simulink model "CAVE_MachE_driver_test"  (R2024a)
settings: configuration reference "ConfigSetDesktopFixedStep" (kept outside this file)
PreLoadFcn:
  | VSS_BICYCLE=Simulink.Variant('Dual=0');
  | VSS_DUAL=Simulink.Variant('Dual=1');
  | Dual=1;
  | load('DriveCycle2.mat')
PostLoadFcn:
  | if any(exist('dsrtsu_mdlpostloadfcn', 'file') ~= 0), dsrtsu_mdlpostloadfcn('Execute', bdroot); end
InitFcn:
  | , if any(exist('rtifpga_mdlclblib', 'file') ~= 0), rtifpga_mdlclblib('Init', bdroot); end,
  | , if any(exist('dsmpb_private', 'file') ~= 0), dsmpb_private('dsmpb_mdlclblib', 'Init', bdroot); end,
  | load('DriveCycle2.mat')
model workspace (MAT data in the model file):
  Gas = 0.383333333333
values from neighbouring files (symbols this model uses):
  CoastDown =     [Run_Simulink.mat]
  limitedMCT =     [Run_Simulink.mat]
  MCT =     [Run_Simulink.mat]
  optimized_speed = [6.8451519807e-19 6.71455685751e-19 6.61817305122e-19 6.79712455505e-19 6.66916107161e-19 6.93956205717e-19 6.71488581248e-19 6.61948887111e-19 6.81653289829e-19 6.68560882013e-19 6.9214695338e-19 6.73330729082e-19 ... (16417 elements, 16417x1)]    [OptimizedSpeed.mat]
  optimized_speed_time = [0 0.1 0.2 0.3 0.4 0.5 0.6 0.7 0.8 0.9 1 1.1 ... (16417 elements, 16417x1)]    [OptimizedSpeed.mat]
  pMCT =     [Run_Simulink.mat]
  RealSimPara =     [Run_Simulink.mat]
  Ref_speed = [13 13.007895099 13.015778396 13.023649891 13.031509584 13.039357475 13.047193564 13.055017851 13.062830336 13.070631019 13.0784199 13.086196979 ... (2669 elements, 2669x1)]    [Ref_speed_and_time.mat]
  Ref_time = [0 0.01 0.02 0.03 0.04 0.05 0.06 0.07 0.08 0.09 0.1 0.11 ... (2669 elements, 2669x1)]    [Ref_speed_and_time.mat]
  US06 =     [Run_Simulink.mat]
undefined symbols (not defined in the file or in its folder): AccelCmd, ActTqLF_Nm_, ActTqLR_Nm_, ActTqRF_Nm_, ActTqRR_Nm_, BattChargeLimitMaxPwr, BattChargeLimitSocBpts, BattChargeLimitTbl, BattChrgCapcty, BattDischargeLimitSocBpts, BattDischargeLimitTbl, BattDischargeMaxPwr, BattNumCellsParallel, BattNumCellsSeries, BattOpenVoltCapBpts, BattOpenVoltTbl, BattResistSocBpts, BattResistTbl, BattResistTempBpts, BrakeMaxPrs, BrakeMaxTrq, ChassisDistCg2FrontAxle, ChassisDistCg2RearAxle, ChassisVehMass, CltchCmd, DecelCmd, DiffRatio, DiscIntNeverNeededParam, EnvGravCnst, EnvPrs, EnvTemp, FuelSpecificGrav, GearCmd, h, InitStates, lgSw, MtrEffSpdBpts, MtrEffTbl, MtrEffTrqBpts, MtrPwrMax, MtrTrqMax, ResultsDrivingTests, SteeringCmd, SupvsryCtrlRegenBrkCutOffTbl, SupvsryCtrlRegenSpdBpts, TestScnrioCycleNum, VEH
libraries: simulink x122, VSIGenLib x122, etargetslib x75, dsmpblib x55, vehdynlibtire x24, autolibshared x22, CarMaker4SL x20, vehdynlibsuspension x14, vehdynlibtirecommon x14, autolibutils x10, VsrLibWheel x8, autolibpowerinfoutils x6
(part 16 of 32)

== system CAVE_MachE_driver_test/Vehicle Under Test3/Vehicle/Driver and Drive Cycle/Driver and PI with FF Control/Speed controller set/Predictive ==
  RefSpd [km/hr] : Inport
  In2 : Inport  Port=2
  Compare To Constant1 : simulink/Logic and Bit Operations/Compare To Constant  relop=<=  const=0.1  OutDataTypeStr=boolean  ZeroCross=off
  Constant : Constant  Value=0
  Constant1 : Constant  Value=0
  Gain : Gain  Gain=1/3.6
  Gain1 : Gain  Gain=1/3.6
  Gain4 : Gain  Gain=100
  Gain5 : Gain  Gain=100
  Longitudinal Driver : autolibshared/Longitudinal Driver  extAccelOvr=off  extDecelOvr=off  extAccelHld=off  extDecelHld=off  extAccelZero=off  extDecelZero=off  cntrlType=Predictive  shftType=None  velUnits=m/s  gearOut=off  Kp=10  Ki=5  Kff=.1  Kg=0  VehVelVec=[0 100]  KffVec=[.1 .1]  KpVec=[10 10]  KiVec=[5 5]  KgVec=[0 0]  m=2040  Kpt=6500  tau=0.1  L=3  aR=200/10  bR=2.5/100  cR=.3  g=9.807  vnom=5  Kaw=1  tauerr=.01  tauPt=2  GearInit=0  tShift=.1  pdlVec=[0.1 0.4 0.5 0.9]  upShftTbl=[-1 12.9375 26.4375 39.9375 51.18749999999999 62.4375 72.84375 83.25;-1 16.3125 29.8125 43.3125 54.5624 65.8125 76.78125 87.75;-1 19.6875 33.1875 46.68749999999999 57.9375 69.1875 80.71875 92.25;-1 33 52.5 77.25 100.5 138.75 161.875 185]  dwnShftTbl=[1 9.5625 23.0625 36.5625 47.8125 59.0625 68.90625 78.75;1 12.9375 26.4375 39.9375 51.18749999999999 62.4375 72.84375 83.25;1 16.3125 29.8125 43.3125 54.562499 65.8125 76.78125 87.75;1 19.6875 33.1875 46.68749999999999 57.9375 69.1875 80.71875 92.25]  tClutch=.5  tRev=.5  tPark=120  aMode=2  UpGearVec="[0  1  2  3  4  5  6  7]"  DownGearVec="[1  2  3  4  5  6  7  8]"
      settings: LibrarySourceBlock=vehdynlibdriver/Longitudinal Driver
  Lowpass Filter : TransferFcn  Denominator=[.02 1]
  Min threshold for Brake switch : Constant  Value=0
  Relational Operator : RelationalOperator  Operator=>  OutDataTypeStr=boolean  InputSameDT=off
  Switch3 : Switch  Criteria=u2 > Threshold  SaturateOnIntegerOverflow=off  InputSameDT=off
  Switch4 : Switch  Criteria=u2 > Threshold  SaturateOnIntegerOverflow=off  InputSameDT=off
  Terminator : Terminator
  standstill brake [0,1] : Constant  Value=0.5
  AccelPedalCmd : Outport
  BrakePedalCmd : Outport  Port=2
  Out3 : Outport  Port=3
  wires:
  Gain1/1 -> Longitudinal Driver/2
  Min threshold for Brake switch/1 -> Relational Operator/2
  Relational Operator/1 -> Out3/1  "BrakeSwitch"
  Constant1/1 -> Longitudinal Driver/3
  RefSpd [km/hr]/1 -> Gain/1
  In2/1 -> Lowpass Filter/1
  Longitudinal Driver/1 -> Terminator/1
  standstill brake [0,1]/1 -> Switch4/1
  Longitudinal Driver/3 -> Switch4/3, Relational Operator/1  "BrakePedalPosPre_pct"
  Switch4/1 -> Gain5/1  "BrakePedalPos_pct"
  Switch3/1 -> Gain4/1  "AcceleratorPedalPos_pct"
  Compare To Constant1/1 -> Switch4/2, Switch3/2
  Constant/1 -> Switch3/1
  Gain4/1 -> AccelPedalCmd/1  "AccelPedalCmd"
  Gain/1 -> Compare To Constant1/1, Longitudinal Driver/1
  Gain5/1 -> BrakePedalCmd/1  "BrakePedalCmd"
  Longitudinal Driver/2 -> Switch3/3  "AcceleratorPedalPosPre_pct"
  Lowpass Filter/1 -> Gain1/1  "VS_Flt"

== system CAVE_MachE_driver_test/Vehicle Under Test3/Vehicle/Driver and Drive Cycle/Driver and PI with FF Control/Speed controller set/Speed tracking controller ==
  RefSpd [km/hr] : Inport
  In2 : Inport  Port=2
  In-house CAVE : Subsystem  VariantControl=varaint1
  PIF : Subsystem  VariantControl=varaint2
  Predictive : Subsystem  VariantControl=varaint3
  AccelPedalCmd : Outport
  BrakePedalCmd : Outport  Port=2
  Out3 : Outport  Port=3

== system CAVE_MachE_driver_test/Vehicle Under Test3/Vehicle/Powertrain Supervisory Controller /Engine Torque Command/Accel Pedal to Traction Wheel Torque Request1/Max Motor Torque ==
  MtrSpd : Inport
  Constant : Constant  Value=MtrPwrMax
  Divide : Product  Inputs=*/
  Saturation : Saturate  UpperLimit=MtrTrqMax  LowerLimit=0
  Saturation1 : Saturate  UpperLimit=inf  LowerLimit=1
  MtrTrqMax : Outport
  wires:
  Saturation/1 -> MtrTrqMax/1
  Saturation1/1 -> Divide/2
  Divide/1 -> Saturation/1
  MtrSpd/1 -> Saturation1/1
  Constant/1 -> Divide/1

== system CAVE_MachE_driver_test/Vehicle Under Test3/Vehicle/Powertrain Supervisory Controller /Engine Torque Command/Motor Torque Arbitration and Power Management/Power Management ==
  note: Power Management algorithm:
      | - Estimate Elec power based on mech power using efficiency map
      | - Check if Elec power is within battery power limits
      | - If power within limit , use motor torque command
      | - If power limit exceeded, use limited motor torque
      | - For low Mot Spd, MotPwrReq will be a small number.  Pass through torque command until Mot Spd > 2.
  BattPwrDischrgLmt : Inport
  BattPwrChrgLmt : Inport  Port=2
  MotSpd : Inport  Port=3
  MotTrqCmd : Inport  Port=4
  Abs : Abs  SaturateOnIntegerOverflow=off
  Check Within Limits : Subsystem
  Compare To Constant : simulink/Logic and Bit Operations/Compare To Constant  relop=<  const=2  OutDataTypeStr=boolean
  ElecToMechPwr : Product  Inputs=*/
  Mech to Elec Power Estimate : Subsystem
  MechPwrToTrq : Product  Inputs=*/
  Switch : Switch  Criteria=u2 > Threshold  SaturateOnIntegerOverflow=off  InputSameDT=off
  Switch1 : Switch  Criteria=u2 > Threshold  SaturateOnIntegerOverflow=off  InputSameDT=off
  Torque Limit : Subsystem
  div0protect - poly : autolibutils/div0protect - poly  thresh=2  ZeroCross1=on  aMode=aMode
  MotTrqCmdFinal : Outport  VectorParamsAs1DForOutWhenUnconnected=off
  wires:
  Compare To Constant/1 -> Switch1/2
  Abs/1 -> Compare To Constant/1
  Switch1/1 -> Torque Limit/1(MotTrq)
  Check Within Limits/1(InLimit) -> Switch/2
  Switch/1 -> Switch1/3
  Check Within Limits/2(y) -> ElecToMechPwr/1
  BattPwrChrgLmt/1 -> Check Within Limits/3(lo)
  Mech to Elec Power Estimate/1(MotPwrElecReq) -> Check Within Limits/2(u)
  BattPwrDischrgLmt/1 -> Check Within Limits/1(up)
  Torque Limit/1(MotTrqCmd) -> MotTrqCmdFinal/1
  MechPwrToTrq/1 -> Switch/3
  ElecToMechPwr/1 -> MechPwrToTrq/1
  Mech to Elec Power Estimate/2(Eff2k) -> ElecToMechPwr/2
  div0protect - poly/1 -> MechPwrToTrq/2
  MotTrqCmd/1 -> Mech to Elec Power Estimate/1(MotTrqCmd), Switch1/1, Switch/1
  MotSpd/1 -> Abs/1, Mech to Elec Power Estimate/2(MotSpd), div0protect - poly/1, Torque Limit/2(MotSpd)

== system CAVE_MachE_driver_test/Vehicle Under Test3/Vehicle/Rototest and ORNL Interface/From Rototest/RotoTestEthRX/Depacker ==
  SysStsBits : Inport
  Extract Bits1 : simulink/Logic and Bit Operations/Extract Bits  bitsToExtract=Range of bits  numBits=8  bitIdxRange=[7]  outScalingMode=Preserve fixed-point scaling
  Extract Bits10 : simulink/Logic and Bit Operations/Extract Bits  bitsToExtract=Range of bits  numBits=8  bitIdxRange=[9]  outScalingMode=Preserve fixed-point scaling
  Extract Bits11 : simulink/Logic and Bit Operations/Extract Bits  bitsToExtract=Range of bits  numBits=8  bitIdxRange=[10]  outScalingMode=Preserve fixed-point scaling
  Extract Bits12 : simulink/Logic and Bit Operations/Extract Bits  bitsToExtract=Range of bits  numBits=8  bitIdxRange=[11]  outScalingMode=Preserve fixed-point scaling
  Extract Bits13 : simulink/Logic and Bit Operations/Extract Bits  bitsToExtract=Range of bits  numBits=8  bitIdxRange=[12]  outScalingMode=Preserve fixed-point scaling
  Extract Bits14 : simulink/Logic and Bit Operations/Extract Bits  bitsToExtract=Range of bits  numBits=8  bitIdxRange=[13]  outScalingMode=Preserve fixed-point scaling
  Extract Bits15 : simulink/Logic and Bit Operations/Extract Bits  bitsToExtract=Range of bits  numBits=8  bitIdxRange=[14]  outScalingMode=Preserve fixed-point scaling
  Extract Bits16 : simulink/Logic and Bit Operations/Extract Bits  bitsToExtract=Range of bits  numBits=8  bitIdxRange=[15]  outScalingMode=Preserve fixed-point scaling
  Extract Bits2 : simulink/Logic and Bit Operations/Extract Bits  bitsToExtract=Range of bits  numBits=8  bitIdxRange=[6]  outScalingMode=Preserve fixed-point scaling
  Extract Bits3 : simulink/Logic and Bit Operations/Extract Bits  bitsToExtract=Range of bits  numBits=8  bitIdxRange=[5]  outScalingMode=Preserve fixed-point scaling
  Extract Bits4 : simulink/Logic and Bit Operations/Extract Bits  bitsToExtract=Range of bits  numBits=8  bitIdxRange=[4]  outScalingMode=Preserve fixed-point scaling
  Extract Bits5 : simulink/Logic and Bit Operations/Extract Bits  bitsToExtract=Range of bits  numBits=8  bitIdxRange=[3]  outScalingMode=Preserve fixed-point scaling
  Extract Bits6 : simulink/Logic and Bit Operations/Extract Bits  bitsToExtract=Range of bits  numBits=8  bitIdxRange=[2]  outScalingMode=Preserve fixed-point scaling
  Extract Bits7 : simulink/Logic and Bit Operations/Extract Bits  bitsToExtract=Range of bits  numBits=8  bitIdxRange=[1]  outScalingMode=Preserve fixed-point scaling
  Extract Bits8 : simulink/Logic and Bit Operations/Extract Bits  bitsToExtract=Range of bits  numBits=8  bitIdxRange=[0]  outScalingMode=Preserve fixed-point scaling
  Extract Bits9 : simulink/Logic and Bit Operations/Extract Bits  bitsToExtract=Range of bits  numBits=8  bitIdxRange=[8]  outScalingMode=Preserve fixed-point scaling
  Gain : Gain  Gain=1/128
  Gain1 : Gain  Gain=1/64
  Gain10 : Gain  Gain=1/1024
  Gain11 : Gain  Gain=1/2048
  Gain12 : Gain  Gain=1/4096
  Gain13 : Gain  Gain=1/8192
  Gain14 : Gain  Gain=1/16384
  Gain15 : Gain  Gain=1/32768
  Gain2 : Gain  Gain=1/32
  Gain3 : Gain  Gain=1/16
  Gain4 : Gain  Gain=1/8
  Gain5 : Gain  Gain=1/4
  Gain6 : Gain  Gain=1/2
  Gain7 : Gain  Gain=1/1
  Gain8 : Gain  Gain=1/256
  Gain9 : Gain  Gain=1/512
  Header : VSIGenLib/Header  not=''
  Terminator{,1..8} (9 alike) : Terminator
  FaultActive : Outport
  WarningsActive : Outport  Port=2
  SpTqRR : Outport  Port=3
  SpTqLR : Outport  Port=4
  SpTqRF : Outport  Port=5
  SpTqLF : Outport  Port=6
  SystemActive : Outport  Port=7
  wires:
  Gain5/1 -> Terminator3/1  "Reserved"
  Gain6/1 -> Terminator4/1  "Reserved"
  Gain3/1 -> Terminator1/1  "Reserved"
  Gain4/1 -> Terminator2/1  "Reserved"
  Gain2/1 -> Terminator/1  "Reserved"
  Gain1/1 -> WarningsActive/1  "WarningsActive"
  Gain/1 -> FaultActive/1  "FaultActive"
  Gain7/1 -> Terminator5/1  "Reserved"
  Gain8/1 -> SystemActive/1  "SystemActive"
  Gain9/1 -> SpTqLF/1  "SpTqLF"
  Gain10/1 -> SpTqRF/1  "SpTqRF"
  Gain11/1 -> SpTqLR/1  "SpTqLR"
  Gain12/1 -> SpTqRR/1  "SpTqRR"
  Gain14/1 -> Terminator7/1  "Reserved"
  Gain13/1 -> Terminator8/1  "Reserved"
  Gain15/1 -> Terminator6/1  "Reserved"
  SysStsBits/1 -> Extract Bits9/1, Extract Bits10/1, Extract Bits16/1, Extract Bits15/1, Extract Bits14/1, Extract Bits13/1, Extract Bits12/1, Extract Bits11/1, Extract Bits8/1, Extract Bits7/1, Extract Bits6/1, Extract Bits5/1, Extract Bits4/1, Extract Bits3/1, Extract Bits2/1, Extract Bits1/1
  Extract Bits16/1 -> Gain15/1
  Extract Bits14/1 -> Gain13/1
  Extract Bits15/1 -> Gain14/1
  Extract Bits13/1 -> Gain12/1
  Extract Bits12/1 -> Gain11/1
  Extract Bits11/1 -> Gain10/1
  Extract Bits9/1 -> Gain8/1
  Extract Bits10/1 -> Gain9/1
  Extract Bits2/1 -> Gain1/1
  Extract Bits5/1 -> Gain4/1
  Extract Bits1/1 -> Gain/1
  Extract Bits3/1 -> Gain2/1
  Extract Bits7/1 -> Gain6/1
  Extract Bits8/1 -> Gain7/1
  Extract Bits4/1 -> Gain3/1
  Extract Bits6/1 -> Gain5/1

== system CAVE_MachE_driver_test/Vehicle Under Test3/Vehicle/Rototest and ORNL Interface/Get Wheel Spd Cmd Based on Wheel Dynamics/Whl Dynamics & Format CM Powertrain Signal/Diff Trq ==
  In1 : Inport
  Constant : Constant  Value=4.1
  Gain10 : Gain  Gain=0.5
  Product : Product  RndMeth=Zero
  Out1 : Outport
  wires:
  Gain10/1 -> Out1/1
  Constant/1 -> Product/1
  In1/1 -> Product/2
  Product/1 -> Gain10/1  "DiffTrq"

== system CAVE_MachE_driver_test/Vehicle Under Test3/Vehicle/Rototest and ORNL Interface/Get Wheel Spd Cmd Based on Wheel Dynamics/Whl Dynamics & Format CM Powertrain Signal/Subsystem ==
  BrakeTorq : Inport
  <Car Trq_T2WFL> : Inport  Port=2
  AxlTorq : Inport  Port=3
  Fx : Inport  Port=4
  Add1 : Sum  Inputs=--+
  Add2 : Sum  Inputs=-+
  Constant : Constant  Value=0
  Constant9 : Constant  Value=0.3135
  MATLAB Function : MATLAB Function  TreatAsAtomicUnit=on
  Memory : Memory
  Output Damping : Gain  Gain=0  SaturateOnIntegerOverflow=on  OutDataTypeStr=Inherit: Same as input  ParamDataTypeStr=Inherit: Same as input
  Product3 : Product  Inputs=**
  Saturation : Saturate  UpperLimit=inf  LowerLimit=0  ZeroCross=off
  Sum : Sum  Inputs=--
  Sum3 : Sum  Inputs=-++
  Switch : Switch  Criteria=u2 > Threshold  SaturateOnIntegerOverflow=off  InputSameDT=off
  WheelInertia : Subsystem
  WheelInertia1 : Subsystem
  omega wheel : Integrator  ContinuousStateAttributes='omegaWheel'
  rotv FL : Outport
  wires:
  Sum3/1 -> WheelInertia/1(In1)
  BrakeTorq/1 -> Sum3/1
  MATLAB Function/1(switchFlag) -> Switch/2  "Flag1"
  Constant/1 -> Switch/1
  Memory/1 -> MATLAB Function/2(wheelSpd)
  Add2/1 -> Saturation/1
  [RhoZ1] -> Add2/1
  Constant9/1 -> Add2/2
  AxlTorq/1 -> Add1/1, MATLAB Function/1(axleTorq), Sum3/3
  <Car Trq_T2WFL>/1 -> Add1/2, Sum3/2
  Product3/1 -> Add1/3
  Saturation/1 -> Product3/2
  Add1/1 -> WheelInertia1/1(In1)
  Switch/1 -> omega wheel/1
  omega wheel/1 -> Memory/1, Output Damping/1, rotv FL/1
  Output Damping/1 -> Sum/2
  WheelInertia1/1(axleTorq) -> Sum/1  "rota"
  Sum/1 -> Switch/3
  [Fx1] -> Product3/1

== system CAVE_MachE_driver_test/Vehicle Under Test3/Vehicle/Rototest and ORNL Interface/Get Wheel Spd Cmd Based on Wheel Dynamics/Whl Dynamics & Format CM Powertrain Signal/Subsystem1 ==
  BrakeTorq : Inport
  <Car Trq_T2WFL> : Inport  Port=2
  AxlTorq : Inport  Port=3
  Discrete-Time Integrator : DiscreteIntegrator  IntegratorMethod=Integration: Backward Euler  InitialCondition=0/3.6/0.3235  SampleTime=0.001  ICPrevOutput=DiscIntNeverNeededParam  ICPrevScaledInput=DiscIntNeverNeededParam
  Sum3 : Sum  Inputs=-++
  WheelInertia : Subsystem
  rotv FL : Outport
  wires:
  Sum3/1 -> WheelInertia/1(In1)
  AxlTorq/1 -> Sum3/3
  <Car Trq_T2WFL>/1 -> Sum3/2
  BrakeTorq/1 -> Sum3/1
  Discrete-Time Integrator/1 -> rotv FL/1  "rotv FL"
  WheelInertia/1(Out1) -> Discrete-Time Integrator/1

== system CAVE_MachE_driver_test/Vehicle Under Test3/Vehicle/Rototest and ORNL Interface/Get Wheel Spd Cmd Based on Wheel Dynamics/Whl Dynamics & Format CM Powertrain Signal/Subsystem2 ==
  BrakeTorq : Inport
  <Car Trq_T2WFR> : Inport  Port=2
  AxlTorq : Inport  Port=3
  Fx : Inport  Port=4
  Add1 : Sum  Inputs=--+
  Add2 : Sum  Inputs=-+
  Constant : Constant  Value=0
  Constant9 : Constant  Value=0.3135
  MATLAB Function : MATLAB Function  TreatAsAtomicUnit=on
  Memory : Memory
  Output Damping : Gain  Gain=-1  SaturateOnIntegerOverflow=on  OutDataTypeStr=Inherit: Same as input  ParamDataTypeStr=Inherit: Same as input
  Product3 : Product  Inputs=**
  Saturation : Saturate  UpperLimit=inf  LowerLimit=0  ZeroCross=off
  Sum3 : Sum  Inputs=-++
  Switch : Switch  Criteria=u2 > Threshold  SaturateOnIntegerOverflow=off  InputSameDT=off
  WheelInertia : Subsystem
  WheelInertia1 : Subsystem
  omega wheel : Integrator  ContinuousStateAttributes='omegaWheel'
  rotv FR : Outport
  wires:
  MATLAB Function/1(switchFlag) -> Switch/2
  Constant/1 -> Switch/1
  BrakeTorq/1 -> Sum3/1
  Sum3/1 -> WheelInertia/1(In1)
  Memory/1 -> MATLAB Function/2(wheelSpd)
  WheelInertia1/1(Out1) -> Output Damping/1  "rota"
  Product3/1 -> Add1/3
  <Car Trq_T2WFR>/1 -> Add1/2, Sum3/2
  Constant9/1 -> Add2/2
  Add1/1 -> WheelInertia1/1(In1)
  [RhoZ2] -> Add2/1
  Saturation/1 -> Product3/2
  Add2/1 -> Saturation/1
  AxlTorq/1 -> Add1/1, MATLAB Function/1(axleTorq), Sum3/3
  omega wheel/1 -> Memory/1, rotv FR/1
  Switch/1 -> omega wheel/1
  Output Damping/1 -> Switch/3
  [Fx2] -> Product3/1

== system CAVE_MachE_driver_test/Vehicle Under Test3/Vehicle/Rototest and ORNL Interface/Get Wheel Spd Cmd Based on Wheel Dynamics/Whl Dynamics & Format CM Powertrain Signal/Subsystem3 ==
  BrakeTorq : Inport
  <Car Trq_T2WRL> : Inport  Port=2
  AxlTorq : Inport  Port=3
  Fx : Inport  Port=4
  FWSpd : Inport  Port=5
  Add1 : Sum  Inputs=--+
  Add2 : Sum  Inputs=-+
  Constant : Constant  Value=0
  Constant9 : Constant  Value=0.3135
  MATLAB Function : MATLAB Function  TreatAsAtomicUnit=on
  Memory : Memory
  Output Damping : Gain  Gain=0  SaturateOnIntegerOverflow=on  OutDataTypeStr=Inherit: Same as input  ParamDataTypeStr=Inherit: Same as input
  Product3 : Product  Inputs=**
  Saturation : Saturate  UpperLimit=inf  LowerLimit=0  ZeroCross=off
  Sum : Sum  Inputs=--
  Sum3 : Sum  Inputs=-++
  Switch : Switch  Criteria=u2 > Threshold  SaturateOnIntegerOverflow=off  InputSameDT=off
  WheelInertia : Subsystem
  WheelInertia1 : Subsystem
  omega wheel : Integrator  ContinuousStateAttributes='omegaWheel'
  rotv RL : Outport
  wires:
  MATLAB Function/1(switchFlag) -> Switch/2
  Constant/1 -> Switch/1
  BrakeTorq/1 -> Sum3/1
  Sum3/1 -> WheelInertia/1(In1)
  Product3/1 -> Add1/3
  <Car Trq_T2WRL>/1 -> Sum3/2, Add1/2
  Constant9/1 -> Add2/2
  Add1/1 -> WheelInertia1/1(In1)
  [RhoZ3] -> Add2/1
  Saturation/1 -> Product3/2
  Add2/1 -> Saturation/1
  AxlTorq/1 -> Add1/1, MATLAB Function/1(axleTorq), Sum3/3
  FWSpd/1 -> MATLAB Function/2(wheelSpd)
  Sum/1 -> Switch/3
  Switch/1 -> omega wheel/1
  [Fx3] -> Product3/1
  Output Damping/1 -> Sum/2
  omega wheel/1 -> Output Damping/1, rotv RL/1
  WheelInertia1/1(axleTorq) -> Sum/1  "rota"

== system CAVE_MachE_driver_test/Vehicle Under Test3/Vehicle/Rototest and ORNL Interface/Get Wheel Spd Cmd Based on Wheel Dynamics/Whl Dynamics & Format CM Powertrain Signal/Subsystem4 ==
  BrakeTorq : Inport
  <Car Trq_T2WRR> : Inport  Port=2
  AxlTorq : Inport  Port=3
  Fx : Inport  Port=4
  FWSpd : Inport  Port=5
  Add1 : Sum  Inputs=--+
  Add2 : Sum  Inputs=-+
  Constant : Constant  Value=0
  Constant9 : Constant  Value=0.3135
  Gain : Gain  Gain=-1
  MATLAB Function : MATLAB Function  TreatAsAtomicUnit=on
  Memory : Memory
  Product3 : Product  Inputs=**
  Saturation : Saturate  UpperLimit=inf  LowerLimit=0  ZeroCross=off
  Sum3 : Sum  Inputs=-++
  Switch : Switch  Criteria=u2 > Threshold  SaturateOnIntegerOverflow=off  InputSameDT=off
  WheelInertia : Subsystem
  WheelInertia1 : Subsystem
  omega wheel : Integrator  ContinuousStateAttributes='omegaWheel'
  rotv RR : Outport
  wires:
  MATLAB Function/1(switchFlag) -> Switch/2
  Constant/1 -> Switch/1
  BrakeTorq/1 -> Sum3/1
  Sum3/1 -> WheelInertia/1(In1)
  Product3/1 -> Add1/3
  <Car Trq_T2WRR>/1 -> Add1/2, Sum3/2
  Constant9/1 -> Add2/2
  Add1/1 -> WheelInertia1/1(In1)
  [RhoZ4] -> Add2/1
  Saturation/1 -> Product3/2
  Add2/1 -> Saturation/1
  AxlTorq/1 -> Add1/1, MATLAB Function/1(axleTorq), Sum3/3
  FWSpd/1 -> MATLAB Function/2(wheelSpd)
  Gain/1 -> Switch/3
  Switch/1 -> omega wheel/1
  omega wheel/1 -> rotv RR/1
  [Fx4] -> Product3/1
  WheelInertia1/1(axleTorq) -> Gain/1  "rota"

== system CAVE_MachE_driver_test/Vehicle Under Test3/Vehicle/Rototest and ORNL Interface/Get Wheel Spd Cmd Based on Wheel Dynamics/Whl Dynamics & Format CM Powertrain Signal/Subsystem5 ==
  In1 : Inport
  <Car Trq_T2WFR> : Inport  Port=2
  In3 : Inport  Port=3
  Discrete-Time Integrator1 : DiscreteIntegrator  IntegratorMethod=Integration: Backward Euler  InitialCondition=0/3.6/0.3235  SampleTime=0.001  ICPrevOutput=DiscIntNeverNeededParam  ICPrevScaledInput=DiscIntNeverNeededParam
  Sum2 : Sum  Inputs=-++
  WheelInertia1 : Subsystem
  rotv FR : Outport
  wires:
  <Car Trq_T2WFR>/1 -> Sum2/2
  Sum2/1 -> WheelInertia1/1(In1)
  In3/1 -> Sum2/3
  WheelInertia1/1(Out1) -> Discrete-Time Integrator1/1  "rota"
  In1/1 -> Sum2/1
  Discrete-Time Integrator1/1 -> rotv FR/1  "rotv FR"

== system CAVE_MachE_driver_test/Vehicle Under Test3/Vehicle/Rototest and ORNL Interface/Get Wheel Spd Cmd Based on Wheel Dynamics/Whl Dynamics & Format CM Powertrain Signal/Subsystem6 ==
  In1 : Inport
  <Car Trq_T2WRL> : Inport  Port=2
  In3 : Inport  Port=3
  Discrete-Time Integrator2 : DiscreteIntegrator  IntegratorMethod=Integration: Backward Euler  InitialCondition=0/3.6/0.3235  SampleTime=0.001  ICPrevOutput=DiscIntNeverNeededParam  ICPrevScaledInput=DiscIntNeverNeededParam
  Sum : Sum  Inputs=-++
  WheelInertia2 : Subsystem
  rotv RL : Outport
  wires:
  In3/1 -> Sum/3
  WheelInertia2/1(Out1) -> Discrete-Time Integrator2/1  "rota"
  <Car Trq_T2WRL>/1 -> Sum/2
  Sum/1 -> WheelInertia2/1(In1)
  Discrete-Time Integrator2/1 -> rotv RL/1  "rotv RL"
  In1/1 -> Sum/1

== system CAVE_MachE_driver_test/Vehicle Under Test3/Vehicle/Rototest and ORNL Interface/Get Wheel Spd Cmd Based on Wheel Dynamics/Whl Dynamics & Format CM Powertrain Signal/Subsystem7 ==
  In1 : Inport
  <Car Trq_T2WRR> : Inport  Port=2
  In3 : Inport  Port=3
  Discrete-Time Integrator3 : DiscreteIntegrator  IntegratorMethod=Integration: Backward Euler  InitialCondition=0/3.6/0.3235  SampleTime=0.001  ICPrevOutput=DiscIntNeverNeededParam  ICPrevScaledInput=DiscIntNeverNeededParam
  Sum1 : Sum  Inputs=-++
  WheelInertia3 : Subsystem
  rotv RR : Outport
  wires:
  Sum1/1 -> WheelInertia3/1(In1)
  WheelInertia3/1(Out1) -> Discrete-Time Integrator3/1  "rota"
  In3/1 -> Sum1/3
  <Car Trq_T2WRR>/1 -> Sum1/2
  In1/1 -> Sum1/1
  Discrete-Time Integrator3/1 -> rotv RR/1  "rotv RR"

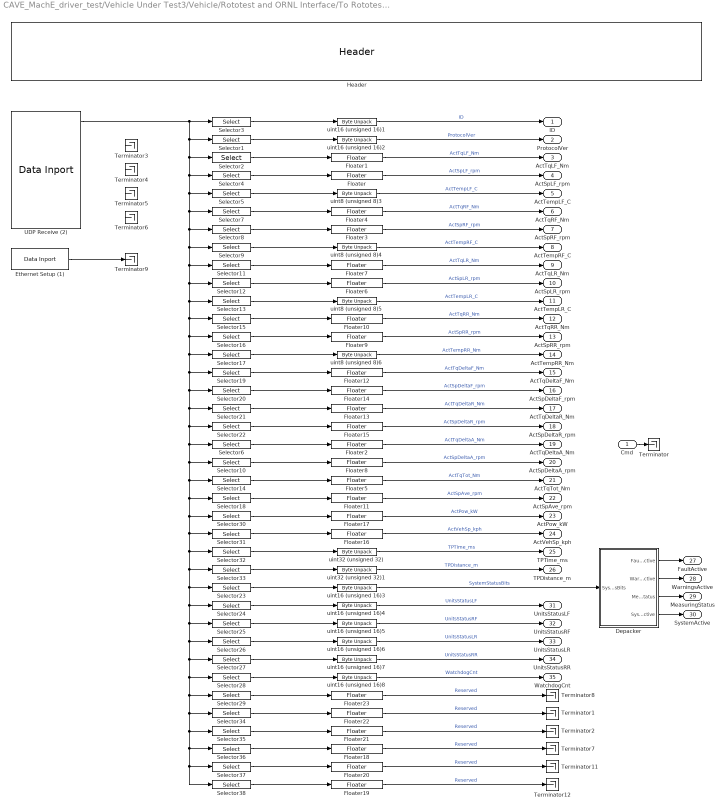
== system CAVE_MachE_driver_test/Vehicle Under Test3/Vehicle/Rototest and ORNL Interface/To Rototest with Band-Aid/Logging/RotoTestEthRXLogging ==
  Cmd : Inport
  Depacker : Subsystem
  Ethernet Setup (1) : dsmpblib/Data Inport  Priority=10000
      settings: SourceProductName=dSPACE Model Interface Package for Simulink (MIPS)
  Floater{,1..23} (24 alike) : VSIGenLib/Floater  SystemSampleTime=-1  VariantActivationTime=update diagram  AllowFlexibleInterface=on  Latency=0  AutoFrameSizeCalculation=off
  Header : VSIGenLib/Header  not=''
  Selector1 : Selector  IndexMode=Zero-based  InputPortWidth=124  IndexOptions=Index vector (dialog)  Indices=[3 2]  OutputSizes=1
  Selector10 : Selector  IndexMode=Zero-based  InputPortWidth=124  IndexOptions=Index vector (dialog)  Indices=[63 62 61 60]  OutputSizes=1
  Selector11 : Selector  IndexMode=Zero-based  InputPortWidth=124  IndexOptions=Index vector (dialog)  Indices=[25 24 23 22]  OutputSizes=1
  Selector12 : Selector  IndexMode=Zero-based  InputPortWidth=124  IndexOptions=Index vector (dialog)  Indices=[29 28 27 26]  OutputSizes=1
  Selector13 : Selector  IndexMode=Zero-based  InputPortWidth=124  IndexOptions=Index vector (dialog)  Indices=[30]  OutputSizes=1
  Selector14 : Selector  IndexMode=Zero-based  InputPortWidth=124  IndexOptions=Index vector (dialog)  Indices=[67 66 65 64]  OutputSizes=1
  Selector15 : Selector  IndexMode=Zero-based  InputPortWidth=124  IndexOptions=Index vector (dialog)  Indices=[34 33 32 31]  OutputSizes=1
  Selector16 : Selector  IndexMode=Zero-based  InputPortWidth=124  IndexOptions=Index vector (dialog)  Indices=[38 37 36 35]  OutputSizes=1
  Selector17 : Selector  IndexMode=Zero-based  InputPortWidth=124  IndexOptions=Index vector (dialog)  Indices=[39]  OutputSizes=1
  Selector18 : Selector  IndexMode=Zero-based  InputPortWidth=124  IndexOptions=Index vector (dialog)  Indices=[71 70 69 68]  OutputSizes=1
  Selector19 : Selector  IndexMode=Zero-based  InputPortWidth=124  IndexOptions=Index vector (dialog)  Indices=[43 42 41 40]  OutputSizes=1
  Selector2 : Selector  IndexMode=Zero-based  InputPortWidth=124  IndexOptions=Index vector (dialog)  Indices=[7 6 5 4]  OutputSizes=1
  Selector20 : Selector  IndexMode=Zero-based  InputPortWidth=124  IndexOptions=Index vector (dialog)  Indices=[47 46 45 44]  OutputSizes=1
  Selector21 : Selector  IndexMode=Zero-based  InputPortWidth=124  IndexOptions=Index vector (dialog)  Indices=[51 50 49 48]  OutputSizes=1
  Selector22 : Selector  IndexMode=Zero-based  InputPortWidth=124  IndexOptions=Index vector (dialog)  Indices=[55 54 53 52]  OutputSizes=1
  Selector23 : Selector  IndexMode=Zero-based  InputPortWidth=124  IndexOptions=Index vector (dialog)  Indices=[89 88]  OutputSizes=1
  Selector24 : Selector  IndexMode=Zero-based  InputPortWidth=124  IndexOptions=Index vector (dialog)  Indices=[91 90]  OutputSizes=1
  Selector25 : Selector  IndexMode=Zero-based  InputPortWidth=124  IndexOptions=Index vector (dialog)  Indices=[93 92]  OutputSizes=1
  Selector26 : Selector  IndexMode=Zero-based  InputPortWidth=124  IndexOptions=Index vector (dialog)  Indices=[95 94]  OutputSizes=1
  Selector27 : Selector  IndexMode=Zero-based  InputPortWidth=124  IndexOptions=Index vector (dialog)  Indices=[97 96]  OutputSizes=1
  Selector28 : Selector  IndexMode=Zero-based  InputPortWidth=124  IndexOptions=Index vector (dialog)  Indices=[99 98]  OutputSizes=1
  Selector29 : Selector  IndexMode=Zero-based  InputPortWidth=124  IndexOptions=Index vector (dialog)  Indices=[103 102 101 100]  OutputSizes=1
  Selector3 : Selector  IndexMode=Zero-based  InputPortWidth=124  IndexOptions=Index vector (dialog)  Indices=[1 0]  OutputSizes=1
  Selector30 : Selector  IndexMode=Zero-based  InputPortWidth=124  IndexOptions=Index vector (dialog)  Indices=[67 66 65 64]  OutputSizes=1
  Selector31 : Selector  IndexMode=Zero-based  InputPortWidth=124  IndexOptions=Index vector (dialog)  Indices=[71 70 69 68]  OutputSizes=1
  Selector32 : Selector  IndexMode=Zero-based  InputPortWidth=124  IndexOptions=Index vector (dialog)  Indices=[83 82 81 80]  OutputSizes=1
  Selector33 : Selector  IndexMode=Zero-based  InputPortWidth=124  IndexOptions=Index vector (dialog)  Indices=[87 86 85 84]  OutputSizes=1
  Selector34 : Selector  IndexMode=Zero-based  InputPortWidth=124  IndexOptions=Index vector (dialog)  Indices=[107 106 105 104]  OutputSizes=1
  Selector35 : Selector  IndexMode=Zero-based  InputPortWidth=124  IndexOptions=Index vector (dialog)  Indices=[111 110 109 108]  OutputSizes=1
  Selector36 : Selector  IndexMode=Zero-based  InputPortWidth=124  IndexOptions=Index vector (dialog)  Indices=[115 114 113 112]  OutputSizes=1
  Selector37 : Selector  IndexMode=Zero-based  InputPortWidth=124  IndexOptions=Index vector (dialog)  Indices=[119 118 117 116]  OutputSizes=1
  Selector38 : Selector  IndexMode=Zero-based  InputPortWidth=124  IndexOptions=Index vector (dialog)  Indices=[123 122 121 120]  OutputSizes=1
  Selector4 : Selector  IndexMode=Zero-based  InputPortWidth=124  IndexOptions=Index vector (dialog)  Indices=[11 10 9 8]  OutputSizes=1
  Selector5 : Selector  IndexMode=Zero-based  InputPortWidth=124  IndexOptions=Index vector (dialog)  Indices=[12]  OutputSizes=1
  Selector6 : Selector  IndexMode=Zero-based  InputPortWidth=124  IndexOptions=Index vector (dialog)  Indices=[59 58 57 56]  OutputSizes=1
  Selector7 : Selector  IndexMode=Zero-based  InputPortWidth=124  IndexOptions=Index vector (dialog)  Indices=[16 15 14 13]  OutputSizes=1
  Selector8 : Selector  IndexMode=Zero-based  InputPortWidth=124  IndexOptions=Index vector (dialog)  Indices=[20 19 18 17]  OutputSizes=1
  Selector9 : Selector  IndexMode=Zero-based  InputPortWidth=124  IndexOptions=Index vector (dialog)  Indices=[21]  OutputSizes=1
  Terminator{,1..9,11..12} (12 alike) : Terminator
  UDP Receive (2) : dsmpblib/Data Inport  Priority=10000
      settings: SourceProductName=dSPACE Model Interface Package for Simulink (MIPS)
  uint16 (unsigned 16){1..8} (8 alike) : etargetslib/Byte Unpack  dimensions={[1]}  datatypes={'uint16'}  byteAlign=1
  uint32 (unsigned 32) : etargetslib/Byte Unpack  dimensions={[1]}  datatypes={'uint32'}  byteAlign=1
  uint32 (unsigned 32)1 : etargetslib/Byte Unpack  dimensions={[1]}  datatypes={'uint32'}  byteAlign=1
  uint8 (unsigned 8){3..6} (4 alike) : etargetslib/Byte Unpack  dimensions={[1]}  datatypes={'uint8'}  byteAlign=1
  ID : Outport
  ProtocolVer : Outport  Port=2
  ActTqLF_Nm : Outport  Port=3
  ActSpLF_rpm : Outport  Port=4
  ActTempLF_C : Outport  Port=5
  ActTqRF_Nm : Outport  Port=6
  ActSpRF_rpm : Outport  Port=7
  ActTempRF_C : Outport  Port=8
  ActTqLR_Nm : Outport  Port=9
  ActSpLR_rpm : Outport  Port=10
  ActTempLR_C : Outport  Port=11
  ActTqRR_Nm : Outport  Port=12
  ActSpRR_rpm : Outport  Port=13
  ActTempRR_Nm : Outport  Port=14
  ActTqDeltaF_Nm : Outport  Port=15
  ActSpDeltaF_rpm : Outport  Port=16
  ActTqDeltaR_Nm : Outport  Port=17
  ActSpDeltaR_rpm : Outport  Port=18
  ActTqDeltaA_Nm : Outport  Port=19
  ActSpDeltaA_rpm : Outport  Port=20
  ActTqTot_Nm : Outport  Port=21
  ActSpAve_rpm : Outport  Port=22
  ActPow_kW : Outport  Port=23
  ActVehSp_kph : Outport  Port=24
  TPTime_ms : Outport  Port=25
  TPDistance_m : Outport  Port=26
  FaultActive : Outport  Port=27
  WarningsActive : Outport  Port=28
  MeasuringStatus : Outport  Port=29
  SystemActive : Outport  Port=30
  UnitsStatusLF : Outport  Port=31
  UnitsStatusRF : Outport  Port=32
  UnitsStatusLR : Outport  Port=33
  UnitsStatusRR : Outport  Port=34
  WatchdogCnt : Outport  Port=35
  wires:
  Selector11/1 -> Floater7/1
  Floater10/1 -> ActTqRR_Nm/1  "ActTqRR_Nm"
  Selector4/1 -> Floater/1
  ? -> Terminator6/1
  Selector1/1 -> uint16 (unsigned 16)2/1
  Selector19/1 -> Floater12/1
  Selector21/1 -> Floater13/1
  Selector28/1 -> uint16 (unsigned 16)8/1
  ? -> Terminator5/1
  Selector3/1 -> uint16 (unsigned 16)1/1
  uint8 (unsigned 8)5/1 -> ActTempLR_C/1  "ActTempLR_C"
  Selector16/1 -> Floater9/1
  Selector15/1 -> Floater10/1
  Selector5/1 -> uint8 (unsigned 8)3/1
  Selector9/1 -> uint8 (unsigned 8)4/1
  Selector20/1 -> Floater14/1
  Floater6/1 -> ActSpLR_rpm/1  "ActSpLR_rpm"
  uint8 (unsigned 8)6/1 -> ActTempRR_Nm/1  "ActTempRR_Nm"
  Selector29/1 -> Floater23/1
  Floater4/1 -> ActTqRF_Nm/1  "ActTqRF_Nm"
  Selector25/1 -> uint16 (unsigned 16)5/1
  ? -> Terminator3/1
  Floater3/1 -> ActSpRF_rpm/1  "ActSpRF_rpm"
  uint16 (unsigned 16)3/1 -> Depacker/1(SysStsBits)  "SystemStatusBits"
  Selector26/1 -> uint16 (unsigned 16)6/1
  Selector13/1 -> uint8 (unsigned 8)5/1
  Selector2/1 -> Floater1/1
  Floater13/1 -> ActTqDeltaR_Nm/1  "ActTqDeltaR_Nm"
  Selector27/1 -> uint16 (unsigned 16)7/1
  uint16 (unsigned 16)4/1 -> UnitsStatusLF/1  "UnitsStatusLF"
  ? -> Terminator4/1
  Selector17/1 -> uint8 (unsigned 8)6/1
  uint16 (unsigned 16)6/1 -> UnitsStatusLR/1  "UnitsStatusLR"
  Selector23/1 -> uint16 (unsigned 16)3/1
  Selector12/1 -> Floater6/1
  Selector22/1 -> Floater15/1
  uint16 (unsigned 16)7/1 -> UnitsStatusRR/1  "UnitsStatusRR"
  Selector8/1 -> Floater3/1
  Selector7/1 -> Floater4/1
  Selector24/1 -> uint16 (unsigned 16)4/1
  uint16 (unsigned 16)2/1 -> ProtocolVer/1  "ProtocolVer"
  Floater7/1 -> ActTqLR_Nm/1  "ActTqLR_Nm"
  Floater12/1 -> ActTqDeltaF_Nm/1  "ActTqDeltaF_Nm"
  uint8 (unsigned 8)3/1 -> ActTempLF_C/1  "ActTempLF_C"
  Floater1/1 -> ActTqLF_Nm/1  "ActTqLF_Nm"
  Floater9/1 -> ActSpRR_rpm/1  "ActSpRR_rpm"
  uint16 (unsigned 16)5/1 -> UnitsStatusRF/1  "UnitsStatusRF"
  Floater14/1 -> ActSpDeltaF_rpm/1  "ActSpDeltaF_rpm"
  uint16 (unsigned 16)8/1 -> WatchdogCnt/1  "WatchdogCnt"
  Floater15/1 -> ActSpDeltaR_rpm/1  "ActSpDeltaR_rpm"
  uint16 (unsigned 16)1/1 -> ID/1  "ID"
  Floater/1 -> ActSpLF_rpm/1  "ActSpLF_rpm"
  uint8 (unsigned 8)4/1 -> ActTempRF_C/1  "ActTempRF_C"
  Depacker/3(MeasuringStatus) -> MeasuringStatus/1
  Depacker/2(WarningsActive) -> WarningsActive/1
  Depacker/1(FaultActive) -> FaultActive/1
  Depacker/4(SystemActive) -> SystemActive/1
  Ethernet Setup (1)/1 -> Terminator9/1
  Floater11/1 -> ActSpAve_rpm/1  "ActSpAve_rpm"
  Floater8/1 -> ActSpDeltaA_rpm/1  "ActSpDeltaA_rpm"
  Floater2/1 -> ActTqDeltaA_Nm/1  "ActTqDeltaA_Nm"
  Selector18/1 -> Floater11/1
  Floater5/1 -> ActTqTot_Nm/1  "ActTqTot_Nm"
  Selector10/1 -> Floater8/1
  Selector14/1 -> Floater5/1
  Selector6/1 -> Floater2/1
  Selector30/1 -> Floater17/1
  Floater17/1 -> ActPow_kW/1  "ActPow_kW"
  Selector31/1 -> Floater16/1
  Floater16/1 -> ActVehSp_kph/1  "ActVehSp_kph"
  uint32 (unsigned 32)/1 -> TPTime_ms/1  "TPTime_ms"
  uint32 (unsigned 32)1/1 -> TPDistance_m/1  "TPDistance_m"
  Selector33/1 -> uint32 (unsigned 32)1/1
  Selector32/1 -> uint32 (unsigned 32)/1
  Selector34/1 -> Floater22/1
  Selector35/1 -> Floater21/1
  Selector36/1 -> Floater18/1
  Selector37/1 -> Floater20/1
  UDP Receive (2)/1 -> Selector3/1, Selector1/1, Selector2/1, Selector4/1, Selector5/1, Selector24/1, Selector28/1, Selector38/1, Selector37/1, Selector36/1, Selector35/1, Selector34/1, Selector29/1, Selector27/1, Selector26/1, Selector25/1, Selector23/1, Selector33/1, Selector32/1, Selector31/1, Selector30/1, Selector18/1, Selector14/1, Selector10/1, Selector6/1, Selector22/1, Selector21/1, Selector20/1, Selector19/1, Selector17/1, Selector16/1, Selector15/1, Selector13/1, Selector12/1, Selector11/1, Selector9/1, Selector8/1, Selector7/1
  Selector38/1 -> Floater19/1
  Floater18/1 -> Terminator7/1  "Reserved"
  Floater19/1 -> Terminator12/1  "Reserved"
  Floater20/1 -> Terminator11/1  "Reserved"
  Floater21/1 -> Terminator2/1  "Reserved"
  Floater22/1 -> Terminator1/1  "Reserved"
  Floater23/1 -> Terminator8/1  "Reserved"
  Cmd/1 -> Terminator/1

== system CAVE_MachE_driver_test/Vehicle Under Test3/Vehicle/Rototest and ORNL Interface/To Rototest with Band-Aid/RotoTestEthTx/Packer ==
  SpTqRR : Inport
  SpTqLR : Inport  Port=2
  SpTqRF : Inport  Port=3
  SpTqLF : Inport  Port=4
  SystemActive : Inport  Port=5
  Add : Sum  Inputs=++++++++  OutDataTypeStr=uint8
  Bit0 : Gain  OutDataTypeStr=uint8
  Bit1 : Gain  Gain=2  OutDataTypeStr=uint8
  Bit2 : Gain  Gain=4  OutDataTypeStr=Inherit: Inherit via back propagation
  Bit3 : Gain  Gain=8  OutDataTypeStr=uint8
  Bit4 : Gain  Gain=16  OutDataTypeStr=uint8
  Bit5 : Gain  Gain=32  OutDataTypeStr=uint8
  Bit6 : Gain  Gain=64  OutDataTypeStr=uint8
  Bit7 : Gain  Gain=128  OutDataTypeStr=uint8
  Ground11 : Ground
  Header : VSIGenLib/Header  not=''
  SystemCtrlBits : Outport
  wires:
  Bit2/1 -> Add/6  "SpTqRF"
  Bit5/1 -> Add/3  "Reserved"
  Ground11/1 -> Bit6/1, Bit5/1, Bit7/1  "Reserved"
  Bit3/1 -> Add/5  "SpTqLR"
  Bit6/1 -> Add/2  "Reserved"
  Bit4/1 -> Add/4  "SpTqRR"
  SystemActive/1 -> Bit0/1
  Bit7/1 -> Add/1  "Reserved"
  Bit1/1 -> Add/7  "SpTqLF"
  Bit0/1 -> Add/8  "SystemActive"
  Add/1 -> SystemCtrlBits/1  "SystemCtrlBits"
  SpTqLR/1 -> Bit3/1
  SpTqRR/1 -> Bit4/1
  SpTqLF/1 -> Bit1/1
  SpTqRF/1 -> Bit2/1

== system CAVE_MachE_driver_test/Vehicle Under Test3/Vehicle/Vehicle Dynamics/Vehicle 14DOF/Subsystem1/Subsystem ==
  Cgxyzdot : Inport
  angles : Inport  Port=2
  Demux2 : Demux  Outputs=3
  Demux3 : Demux  Outputs=3
  Terminator{,1..4} (5 alike) : Terminator
  VehSpd : Outport
  wires:
  Demux2/1 -> VehSpd/1  "xdot"
  angles/1 -> Demux3/1
  Demux2/3 -> Terminator1/1  "zdot"
  Demux3/3 -> Terminator4/1  "psi"
  Demux3/1 -> Terminator2/1  "phi"
  Demux2/2 -> Terminator/1  "xdot"
  Demux3/2 -> Terminator3/1  "theta"
  Cgxyzdot/1 -> Demux2/1

== system CAVE_MachE_driver_test/Vehicle Under Test3/Vehicle/Vehicle Dynamics/Vehicle 14DOF/Subsystem4/Subsystem ==
  Cgxyzdot : Inport
  angles : Inport  Port=2
  Demux2 : Demux  Outputs=3
  Demux3 : Demux  Outputs=3
  Terminator{,1..4} (5 alike) : Terminator
  VehSpd : Outport
  wires:
  Cgxyzdot/1 -> Demux2/1
  Demux3/2 -> Terminator3/1  "theta"
  Demux2/2 -> Terminator/1  "xdot"
  Demux3/1 -> Terminator2/1  "phi"
  Demux3/3 -> Terminator4/1  "psi"
  Demux2/3 -> Terminator1/1  "zdot"
  angles/1 -> Demux3/1
  Demux2/1 -> VehSpd/1  "xdot"

== system CAVE_MachE_driver_test/Vehicle Under Test3/Vehicle/Vehicle Dynamics/Vehicle 14DOF/Suspension/Double Wishbone Suspension ==
  Wheel : Inport
  Steering : Inport  Port=2
  Vehicle : Inport  Port=3
  Bus Creator1 : BusCreator  Inputs=5
  Bus Creator2 : BusCreator  Inputs=2
  Bus Creator3 : BusCreator  Inputs=2
  Bus Creator4 : BusCreator  Inputs=6
  Bus Selector : BusSelector  OutputSignals=z,Re,zdot,Fx,Fy,M
  Bus Selector1 : BusSelector  OutputSignals=P,V
  Independent Suspension – Double Wishbone : vehdynlibsuspension/Independent Suspension - Double Wishbone  ActiveDampEn=off  NumAxl=2  NumWhlsByAxl=[2 2]  StrgEnByAxl=[1 0]  AntiSwayEnByAxl=[1 0]  WhlNumVec="[1  2  1  2]"  AxleNumVec="[1  1  2  2]"  SuspTypesByAxle="[1  1]"  SuspImage=suspdw.png  IdealSuspEn=on  IdealSuspAxles="[1  2]"  Kz=Kz  F0z=F0z  Cz=Cz  Hmax=Hmax  f_act_susp_cz=[10000 10000;10000 10000]  f_act_susp_duty_bpt=[0 1]  f_act_susp_zdot_bpt=[-1 1]  Toe=0.  RollStrgSlp=0.  ToeStrgSlp=0.  Caster=0.  CasterHslp=0.  CasterStrgSlp=0.  Camber=0.  CamberHslp=0.  CamberStrgSlp=0.  StrgHgtSlp=0.1432  MappedSuspEn=off  MappedSuspAxles="[1  2]"  f_susp_axl_bp=[1 2]  f_susp_dz_bp=[-0.15 -0.14 -0.13 -0.12 -0.11 -0.10 -0.09 -0.08 -0.07 -0.06 -0.05 -0.04 -0.03 -0.02 -0.01 0.00 0.01 0.02 0.03 0.04 0.05 0.06 0.07 0.08 0.09 0.10 0.11 0.12 0.13 0.14 0.15]  f_susp_dzdot_bp=[-0.15 -0.14 -0.13 -0.12 -0.11 -0.10 -0.09 -0.08 -0.07 -0.06 -0.05 -0.04 -0.03 -0.02 -0.01 0.00 0.01 0.02 0.03 0.04 0.05 0.06 0.07 0.08 0.09 0.10 0.11 0.12 0.13 0.14 0.15]  f_susp_fmz=zeros(31,31,61,2,4)  f_susp_geom=zeros(31,61,2,3)  f_susp_strgdelta_bp=[-30,-29,-28,-27,-26,-25,-24,-23,-22,-21,-20,-19,-18,-17,-16,-15,-14,-13,-12,-11,-10,-9,-8,-7,-6,-5,-4,-3,-2,-1,0,1,2,3,4,5,6,7,8,9,10,11,12,13,14,15,16,17,18,19,20,21,22,23,24,25,26,27,28,29,30]  AntiSwayR=0.2  AntiSwayNtrlAng=0.5236  AntiSwayTrsK=8e2
  Selector1 : Selector  NumberOfDimensions=2  IndexOptions=Index vector (dialog),Select all  Indices=1,1  OutputSizes=1,1
  Selector2 : Selector  NumberOfDimensions=2  IndexOptions=Index vector (dialog),Select all  Indices=2,1  OutputSizes=1,1
  Steer Rate Adapter : Subsystem
  Steering Adapter : Subsystem
  Terminator : Terminator
  Vehicle Adapter : Subsystem
  Wheel  Adapter : Subsystem
  Suspension : Outport  VectorParamsAs1DForOutWhenUnconnected=off
  wires:
  Bus Creator3/1 -> Suspension/1
  Steering Adapter/1(StrgAng) -> Independent Suspension – Double Wishbone/9
  Independent Suspension – Double Wishbone/1 -> Terminator/1  "Susp"
  Wheel  Adapter/6(Re) -> Bus Creator4/6
  Bus Selector1/1 -> Independent Suspension – Double Wishbone/7  "<P>"
  Wheel  Adapter/2(WhlFy) -> Bus Creator4/2  "Fy"
  Wheel/1 -> Wheel  Adapter/1(Wheels)
  Steer Rate Adapter/1(AngVel) -> Bus Creator1/5  "AngVel"
  Bus Creator4/1 -> Bus Selector/1
  Bus Creator2/1 -> Bus Creator3/1  "Veh"
  Independent Suspension – Double Wishbone/5 -> Selector2/1, Selector1/1  "V"
  Selector2/1 -> Bus Creator1/3  "ydot"
  Bus Selector1/2 -> Independent Suspension – Double Wishbone/8  "<V>"
  Independent Suspension – Double Wishbone/2 -> Bus Creator2/1  "F"
  Bus Selector/2 -> Independent Suspension – Double Wishbone/2  "<Re>"
  Wheel  Adapter/5(M) -> Bus Creator4/5  "M"
  Bus Selector/4 -> Independent Suspension – Double Wishbone/4  "<Fx>"
  Independent Suspension – Double Wishbone/4 -> Bus Creator1/1  "F"
  Steering/1 -> Steering Adapter/1(Steer)
  Selector1/1 -> Bus Creator1/2  "xdot"
  Independent Suspension – Double Wishbone/3 -> Bus Creator2/2  "M"
  Vehicle Adapter/1(VehSusp) -> Bus Selector1/1
  Wheel  Adapter/4(zdot) -> Bus Creator4/4
  Vehicle/1 -> Steer Rate Adapter/1(Veh), Vehicle Adapter/1(Veh)
  Bus Selector/6 -> Independent Suspension – Double Wishbone/6  "<M>"
  Bus Selector/5 -> Independent Suspension – Double Wishbone/5  "<Fy>"
  Bus Selector/1 -> Independent Suspension – Double Wishbone/1  "<z>"
  Wheel  Adapter/3(z) -> Bus Creator4/3
  Independent Suspension – Double Wishbone/6 -> Bus Creator1/4  "Ang"
  Bus Creator1/1 -> Bus Creator3/2  "Whl"
  Wheel  Adapter/1(WhlFx) -> Bus Creator4/1  "Fx"
  Bus Selector/3 -> Independent Suspension – Double Wishbone/3  "<zdot>"
